simulink model "SimpleSensorModel"  (R2020b)
settings: Solver=VariableStepAuto  StartTime=0.0  StopTime=5  RelTol=1e-3
libraries: dspfdesign x1, simulink x1
settings Model: Creator=bolic  LastModifiedBy=bolic

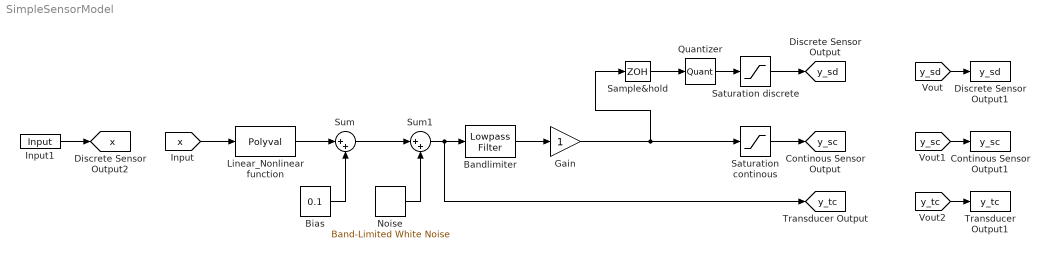
== system SimpleSensorModel ==
  Bandlimiter : dspfdesign/Lowpass Filter  FilterType=FIR  DesignForMinimumOrder=on  FilterOrder=50  PassbandFrequency=100  StopbandFrequency=150  PassbandRipple=0.1  StopbandAttenuation=30  InheritSampleRate=off  SampleRate=10000  SimulateUsing=Interpreted execution  roundingMode=Floor  coeffsDataTypeStr=fixdt(1,16)
  Bias : Constant  Value=0.1  SampleTime=0.0001
  Continous Sensor Output1 : ToWorkspace  VariableName=y_sc  SaveFormat=Timeseries  SampleTime=-1
  Discrete Sensor Output1 : ToWorkspace  VariableName=y_sd  SaveFormat=Timeseries  SampleTime=-1
  Gain : Gain
  Input1 : FromWorkspace  VariableName=Input  SampleTime=0.0001  OutputAfterFinalValue=Setting to zero
  Linear_Nonlinear function : Polyval  Coefs=[-0.015, 0.08,1,0]
  Noise : simulink/Sources/Band-Limited White Noise  Cov=0  Ts=0.0001  seed=[23341]
  Quantizer : Quantizer  QuantizationInterval=5/2^8
  Sample&hold : ZeroOrderHold  SampleTime=1/100
  Saturation continous : Saturate  UpperLimit=5  LowerLimit=0
  Saturation discrete : Saturate  UpperLimit=5  LowerLimit=0
  Sum : Sum  Inputs=|++
  Sum1 : Sum  Inputs=|++
  Transducer Output1 : ToWorkspace  VariableName=y_tc  SaveFormat=Timeseries  SampleTime=-1
  tag scope: x=global, y_sc=global, y_sd=global, y_tc=global
  wires:
  Bandlimiter/1 -> Gain/1
  Linear_Nonlinear function/1 -> Sum/1
  Sum/1 -> Sum1/1
  Noise/1 -> Sum1/2
  Bias/1 -> Sum/2
  [y_sd] -> Discrete Sensor Output1/1
  [y_sc] -> Continous Sensor Output1/1
  Sum1/1 -> [y_tc], Bandlimiter/1
  [y_tc] -> Transducer Output1/1
  Input1/1 -> [x]
  [x] -> Linear_Nonlinear function/1
  Sample&hold/1 -> Quantizer/1
  Quantizer/1 -> Saturation discrete/1
  Saturation continous/1 -> [y_sc]
  Saturation discrete/1 -> [y_sd]
  Gain/1 -> Sample&hold/1, Saturation continous/1
